simulink model "gm_sampleModel1400_5_sub"  (R2023a)
settings: Solver=VariableStepAuto  StartTime=0.0  StopTime=10.0  RelTol=1e-3
libraries: hdlsllib x1, simulink x1
settings Model: Creator=user1  LastModifiedBy=user1
settings OptimizationCC: BlockReduction=off  ConditionallyExecuteInputs=off
settings DebuggingCC: InheritedTsInSrcMsg=none

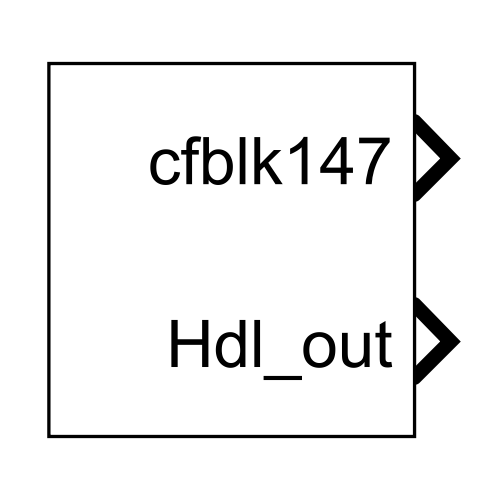
[thumbnail: Simulink's stored preview of the top-level diagram]
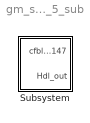
== system gm_sampleModel1400_5_sub ==
  Subsystem : Subsystem

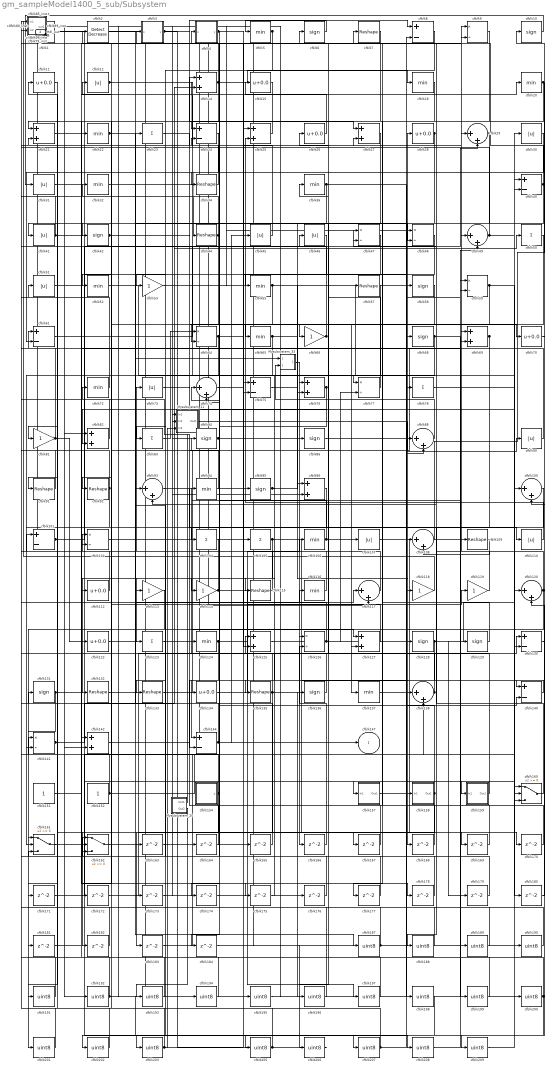
== system gm_sampleModel1400_5_sub/Subsystem ==
  Mysubsystem_11 : Subsystem
  Mysubsystem_20 : Subsystem
  Mysubsystem_33 : Subsystem
  cfblk1 : hdlsllib/Logic and Bit Operations/Bit Slice  lidx=7  ridx=0
  cfblk{6,10,42,58,68,84,86,95,128..129,131,136} (12 alike) : Signum
  cfblk{29,49,74,88,93,100,108,117,120,138} (10 alike) : Sum  Inputs=|++  OutDataTypeStr=uint8
  cfblk{8,24,40,61,75,101,130,140,144} (9 alike) : Sum  Inputs=+-  OutDataTypeStr=uint8
  cfblk{9,47..48,59,64,77,102,126,141} (9 alike) : Product  Inputs=*/  OutDataTypeStr=uint8  RndMeth=Zero  SaturateOnIntegerOverflow=on
  cfblk{23,50,78,83,104..105,123} (7 alike) : Sum  Inputs=+  OutDataTypeStr=uint8
  cfblk{5,18,20,22,32,36,52,55,65,72,94,106,116,124,137} (15 alike) : MinMax  OutDataTypeStr=uint8
  cfblk{12,30..31,41,45..46,51,73,90,107,110} (11 alike) : Abs  OutDataTypeStr=uint8  SaturateOnIntegerOverflow=off
  cfblk{7,34,44,57,91..92,109,115,132..133,135} (11 alike) : Reshape
  cfblk{11,15,26,28,70,112,122,134} (8 alike) : Bias  Bias=0.0  SaturateOnIntegerOverflow=off
  cfblk{53,66,81,113..114,118..119} (7 alike) : Gain  OutDataTypeStr=uint8
  cfblk{14,21,25,27,69,76,82,96,125,127,142} (11 alike) : Sum  OutDataTypeStr=uint8
  cfblk139_inst : Subsystem
  cfblk13_inst : Subsystem
  cfblk143_inst : Subsystem
  cfblk145_inst : Subsystem
  cfblk146_inst : Subsystem
  cfblk151 : Constant  OutDataTypeStr=uint8  SampleTime=-1
  cfblk152 : Constant  OutDataTypeStr=uint8  SampleTime=-1
  cfblk154 : Subsystem  mask(Counter Limited){uplimit=double(7), tsamp=double(-1)}
      mask prompts: uplimit "Simulink:masks:UpperLimit_MP"; tsamp "Simulink:masks:SampleTime_MP"
      mask help: Simulink:masks:CounterLimited_MD
      mask init:
      | nbits = double(8);
      | tsamp = double(-1);
      | uplimit = double(7);
  cfblk157 : Subsystem
  cfblk158 : Subsystem
  cfblk159 : Subsystem
  cfblk160 : Switch  OutDataTypeStr=uint8  SaturateOnIntegerOverflow=off  InputSameDT=off
  cfblk161 : Switch  OutDataTypeStr=uint8  SaturateOnIntegerOverflow=off  InputSameDT=off
  cfblk162 : Switch  OutDataTypeStr=uint8  SaturateOnIntegerOverflow=off  InputSameDT=off
  cfblk{163..184} (22 alike) : Delay  SampleTime=1
  cfblk16_inst : Subsystem
  cfblk17_inst : Subsystem
  cfblk{187..203,205..209} (22 alike) : DataTypeConversion  OutDataTypeStr=uint8  SaturateOnIntegerOverflow=off  RndMeth=Floor
  cfblk19_inst : Subsystem
  cfblk2 : simulink/Logic and Bit Operations/Detect Decrease  vinit=0.0  OutDataTypeStr=uint8
      settings: LibrarySourceBlock=|
      | hdlsllib/Logic and Bit
      | Operations/Detect
      | Decrease
  cfblk3 : Subsystem  mask(Compare To Zero){relop=<=, OutDataTypeStr=uint8, ZeroCross=on}
      mask prompts: relop "Simulink:masks:Operator_MP"; OutDataTypeStr "Simulink:masks:OutputDataType_MP"; ZeroCross "Simulink:masks:EnableZerocrossingDetection_MP"
      mask help: Simulink:masks:CompareToZero_MD
      mask init:
      | OutDataTypeStr = 'uint8';
      | ZeroCross = 'on';
      | blkName = 'sampleModel1400_5_sub/Subsystem/cfblk3';
      | relop = '<=';
      | setValue = 'fixdt(0, 8)';
      mask TypeOptions relop: == | ~= | < | <= | >= | >
      mask TypeOptions OutDataTypeStr: Simulink:masks:uint8 | Simulink:masks:boolean
      mask Callback ZeroCross: sl('zeroCrossEnable', gcbh);
      mask Display: disp([relop,' 0'])
  cfblk35_inst : Subsystem
  cfblk37_inst : Subsystem
  cfblk39_inst : Subsystem
  cfblk4 : Subsystem  mask(Compare To Constant){relop=<=, const=double(3), OutDataTypeStr=uint8, ZeroCross=on}
      mask prompts: relop "Simulink:masks:Operator_MP"; const "Simulink:masks:ConstantValue_MP"; OutDataTypeStr "Simulink:masks:OutputDataType_MP"; ZeroCross "Simulink:masks:EnableZerocrossingDetection_MP"
      mask help: Simulink:masks:CompareToConstant_MD
      mask init:
      | OutDataTypeStr = 'uint8';
      | ZeroCross = 'on';
      | blkName = 'sampleModel1400_5_sub/Subsystem/cfblk4';
      | const = double(3);
      | const_str = '3.0';
      | const_val = double(3);
      | relop = '<=';
      | setValue = 'fixdt(0, 8)';
      | str = '<= 3';
      mask TypeOptions relop: == | ~= | < | <= | >= | >
      mask TypeOptions OutDataTypeStr: Simulink:masks:uint8 | Simulink:masks:boolean
      mask Callback ZeroCross: sl('zeroCrossEnable', gcbh);
      mask Display: disp(str)
  cfblk43_inst : Subsystem
  cfblk54_inst : Subsystem
  cfblk60_inst : Subsystem
  cfblk62_inst : Subsystem
  cfblk67_inst : Subsystem
  cfblk71_inst : Subsystem
  cfblk79_inst : Subsystem
  cfblk80_inst : Subsystem
  cfblk85_inst : Subsystem
  cfblk98_inst : Subsystem
  cfblk99_inst : Subsystem
  cfblk147 : Outport  OutDataTypeStr=uint8  SampleTime=1  VectorParamsAs1DForOutWhenUnconnected=off
  Hdl_out : Outport  Port=2  OutDataTypeStr=uint8  SampleTime=1
  wires:
  Mysubsystem_11/1(Out1) -> cfblk168/1
  Mysubsystem_20/1(Out1) -> cfblk50/1
  Mysubsystem_20/2(Out2) -> cfblk193/1
  Mysubsystem_33/1(Out1) -> cfblk166/1
  cfblk1/1 -> cfblk205/1
  cfblk10/1 -> cfblk31/1
  cfblk100/1 -> cfblk188/1
  cfblk101/1 -> cfblk46/1, cfblk159/1(In1), cfblk157/1(In1)
  cfblk102/1 -> cfblk28/1
  cfblk104/1 -> cfblk132/1
  cfblk105/1 -> cfblk169/1, cfblk123/1
  cfblk106/1 -> cfblk6/1, cfblk4/1(u)
  cfblk107/1 -> cfblk170/1
  cfblk108/1 -> cfblk10/1
  cfblk109/1 -> cfblk108/2
  cfblk11/1 -> cfblk91/1
  cfblk110/1 -> cfblk25/2
  cfblk112/1 -> cfblk61/1
  cfblk113/1 -> cfblk201/1
  cfblk114/1 -> cfblk197/1, cfblk112/1
  cfblk115/1 -> cfblk60_inst/1(in1)
  cfblk116/1 -> cfblk99_inst/1(in1)
  cfblk117/1 -> cfblk73/1
  cfblk118/1 -> cfblk19_inst/2(in2)
  cfblk119/1 -> cfblk93/2
  cfblk12/1 -> cfblk76/1, cfblk44/1
  cfblk120/1 -> cfblk9/1, cfblk47/1, cfblk181/1
  cfblk122/1 -> cfblk116/1
  cfblk123/1 -> cfblk127/1
  cfblk124/1 -> cfblk144/1, cfblk119/1
  cfblk125/1 -> cfblk138/1
  cfblk126/1 -> cfblk71_inst/2(in2), cfblk77/2
  cfblk127/1 -> cfblk102/1
  cfblk128/1 -> cfblk30/1, cfblk144/2, cfblk179/1
  cfblk129/1 -> cfblk3/1(u)
  cfblk13_inst/1(out1) -> cfblk200/1
  cfblk130/1 -> cfblk207/1
  cfblk131/1 -> cfblk7/1, cfblk161/1
  cfblk132/1 -> cfblk94/1
  cfblk133/1 -> cfblk49/1
  cfblk134/1 -> cfblk106/1
  cfblk135/1 -> cfblk62_inst/1(in1), cfblk17_inst/2(in2), cfblk182/1, cfblk158/1(In1)
  cfblk136/1 -> cfblk11/1
  cfblk137/1 -> cfblk128/1
  cfblk138/1 -> cfblk99_inst/2(in2), cfblk12/1
  cfblk139_inst/1(out1) -> cfblk195/1
  cfblk14/1 -> cfblk43_inst/2(in2), cfblk21/1, cfblk18/1
  cfblk140/1 -> cfblk134/1
  cfblk141/1 -> cfblk51/1, cfblk14/2, cfblk23/1
  cfblk142/1 -> cfblk69/1
  cfblk143_inst/1(out1) -> cfblk101/2
  cfblk144/1 -> cfblk98_inst/2(in2), cfblk45/1
  cfblk145_inst/1(out1) -> cfblk95/1, cfblk142/2
  cfblk146_inst/1(out1) -> cfblk192/1
  cfblk15/1 -> cfblk64/2
  cfblk151/1 -> cfblk22/1
  cfblk152/1 -> cfblk35_inst/2(in2), cfblk108/1
  cfblk154/1(y) -> cfblk84/1, cfblk191/1, cfblk141/1
  cfblk157/1(Out1) -> cfblk140/2
  cfblk158/1(Out1) -> cfblk74/1, cfblk183/1
  cfblk159/1(Out1) -> cfblk36/1
  cfblk16_inst/1(out1) -> cfblk117/2
  cfblk160/1 -> cfblk62_inst/2(in2)
  cfblk161/1 -> cfblk175/1
  cfblk162/1 -> cfblk167/1
  cfblk163/1 -> cfblk138/2
  cfblk164/1 -> cfblk101/1
  cfblk165/1 -> cfblk37_inst/1(in1)
  cfblk166/1 -> cfblk126/2
  cfblk167/1 -> cfblk143_inst/2(in2)
  cfblk168/1 -> cfblk47/2
  cfblk169/1 -> cfblk80_inst/2(in2)
  cfblk17_inst/1(out1) -> cfblk165/1
  cfblk170/1 -> cfblk25/1
  cfblk171/1 -> cfblk40/2
  cfblk172/1 -> cfblk49/2
  cfblk173/1 -> cfblk59/2
  cfblk174/1 -> cfblk117/1
  cfblk175/1 -> cfblk125/1
  cfblk176/1 -> cfblk24/2
  cfblk177/1 -> cfblk39_inst/2(in2)
  cfblk178/1 -> cfblk93/1
  cfblk179/1 -> cfblk16_inst/1(in1)
  cfblk18/1 -> cfblk177/1
  cfblk180/1 -> cfblk120/2
  cfblk181/1 -> cfblk69/2
  cfblk182/1 -> cfblk145_inst/1(in1)
  cfblk183/1 -> cfblk8/2
  cfblk184/1 -> cfblk206/1
  cfblk187/1 -> cfblk90/1, cfblk131/1
  cfblk188/1 -> cfblk2/1
  cfblk189/1 -> cfblk79_inst/1(in1)
  cfblk19_inst/1(out1) -> cfblk58/1
  cfblk190/1 -> cfblk67_inst/1(in1)
  cfblk191/1 -> cfblk67_inst/2(in2)
  cfblk192/1 -> cfblk80_inst/1(in1), cfblk208/1
  cfblk193/1 -> cfblk146_inst/1(in1)
  cfblk194/1 -> cfblk146_inst/2(in2)
  cfblk195/1 -> cfblk136/1
  cfblk196/1 -> cfblk139_inst/1(in1)
  cfblk197/1 -> cfblk139_inst/2(in2)
  cfblk198/1 -> cfblk202/1
  cfblk199/1 -> cfblk32/1
  cfblk2/1 -> cfblk187/1
  cfblk20/1 -> cfblk140/1, cfblk52/1
  cfblk200/1 -> cfblk209/1, cfblk142/1
  cfblk201/1 -> cfblk13_inst/1(in1)
  cfblk202/1 -> cfblk13_inst/2(in2)
  cfblk203/1 -> cfblk79_inst/2(in2), cfblk9/2, Mysubsystem_11/3(In3)
  cfblk205/1 -> cfblk39_inst/1(in1), cfblk161/3
  cfblk206/1 -> cfblk1/1
  cfblk207/1 -> cfblk88/2, cfblk162/1
  cfblk208/1 -> cfblk130/1
  cfblk209/1 -> cfblk130/2
  cfblk21/1 -> cfblk178/1
  cfblk22/1 -> cfblk48/2, Mysubsystem_33/1(In1)
  cfblk23/1 -> cfblk77/1
  cfblk24/1 -> cfblk61/2
  cfblk25/1 -> cfblk24/1
  cfblk26/1 -> cfblk15/1
  cfblk27/1 -> cfblk196/1
  cfblk28/1 -> cfblk162/2, Mysubsystem_11/2(In2)
  cfblk29/1 -> cfblk41/1, Mysubsystem_11/1(In1)
  cfblk3/1(y) -> cfblk8/1, cfblk27/1
  cfblk30/1 -> cfblk92/1
  cfblk31/1 -> cfblk173/1
  cfblk32/1 -> cfblk198/1
  cfblk34/1 -> cfblk19_inst/1(in1)
  cfblk35_inst/1(out1) -> cfblk86/1, Hdl_out/1
  cfblk36/1 -> cfblk88/1, cfblk74/2
  cfblk37_inst/1(out1) -> cfblk124/1
  cfblk39_inst/1(out1) -> cfblk129/1, cfblk147/1
  cfblk4/1(y) -> cfblk75/1, cfblk184/1
  cfblk40/1 -> cfblk76/2, cfblk60_inst/2(in2), cfblk81/1
  cfblk41/1 -> cfblk75/2, cfblk17_inst/1(in1), cfblk78/1
  cfblk42/1 -> cfblk70/1, cfblk180/1
  cfblk43_inst/1(out1) -> cfblk176/1
  cfblk44/1 -> cfblk85_inst/2(in2), cfblk163/1
  cfblk45/1 -> cfblk14/1
  cfblk46/1 -> cfblk55/1
  cfblk47/1 -> cfblk126/1
  cfblk48/1 -> cfblk125/2
  cfblk49/1 -> cfblk40/1, cfblk145_inst/2(in2)
  cfblk5/1 -> cfblk34/1, cfblk133/1
  cfblk50/1 -> cfblk203/1
  cfblk51/1 -> cfblk20/1
  cfblk52/1 -> cfblk100/1
  cfblk53/1 -> cfblk27/2
  cfblk54_inst/1(out1) -> cfblk98_inst/1(in1)
  cfblk55/1 -> cfblk160/2, cfblk65/1
  cfblk57/1 -> cfblk135/1
  cfblk58/1 -> cfblk127/2
  cfblk59/1 -> cfblk160/1, cfblk172/1
  cfblk6/1 -> cfblk5/1
  cfblk60_inst/1(out1) -> cfblk190/1
  cfblk61/1 -> cfblk29/2
  cfblk62_inst/1(out1) -> cfblk54_inst/2(in2)
  cfblk64/1 -> cfblk66/1, cfblk171/1
  cfblk65/1 -> cfblk118/1, cfblk83/1
  cfblk66/1 -> cfblk85_inst/1(in1), cfblk16_inst/2(in2)
  cfblk67_inst/1(out1) -> cfblk189/1
  cfblk68/1 -> cfblk199/1, cfblk160/3, cfblk141/2
  cfblk69/1 -> cfblk162/3, cfblk104/1
  cfblk7/1 -> cfblk102/2
  cfblk70/1 -> cfblk100/2
  cfblk71_inst/1(out1) -> cfblk194/1
  cfblk72/1 -> cfblk37_inst/2(in2)
  cfblk73/1 -> cfblk137/1
  cfblk74/1 -> cfblk29/1
  cfblk75/1 -> cfblk96/1
  cfblk76/1 -> cfblk82/2, cfblk113/1
  cfblk77/1 -> cfblk26/1
  cfblk78/1 -> cfblk120/1
  cfblk79_inst/1(out1) -> cfblk48/1
  cfblk8/1 -> cfblk53/1
  cfblk80_inst/1(out1) -> cfblk107/1, cfblk105/1
  cfblk81/1 -> cfblk71_inst/1(in1), cfblk21/2, cfblk122/1
  cfblk82/1 -> cfblk43_inst/1(in1)
  cfblk83/1 -> cfblk64/1
  cfblk84/1 -> cfblk68/1, cfblk114/1
  cfblk85_inst/1(out1) -> cfblk164/1
  cfblk86/1 -> cfblk59/1
  cfblk88/1 -> Mysubsystem_33/2(In2)
  cfblk9/1 -> cfblk42/1
  cfblk90/1 -> cfblk54_inst/1(in1)
  cfblk91/1 -> cfblk143_inst/1(in1)
  cfblk92/1 -> cfblk35_inst/1(in1), cfblk161/2
  cfblk93/1 -> cfblk110/1
  cfblk94/1 -> cfblk72/1
  cfblk95/1 -> cfblk57/1, cfblk115/1
  cfblk96/1 -> cfblk174/1
  cfblk98_inst/1(out1) -> cfblk96/2, cfblk109/1
  cfblk99_inst/1(out1) -> cfblk82/1

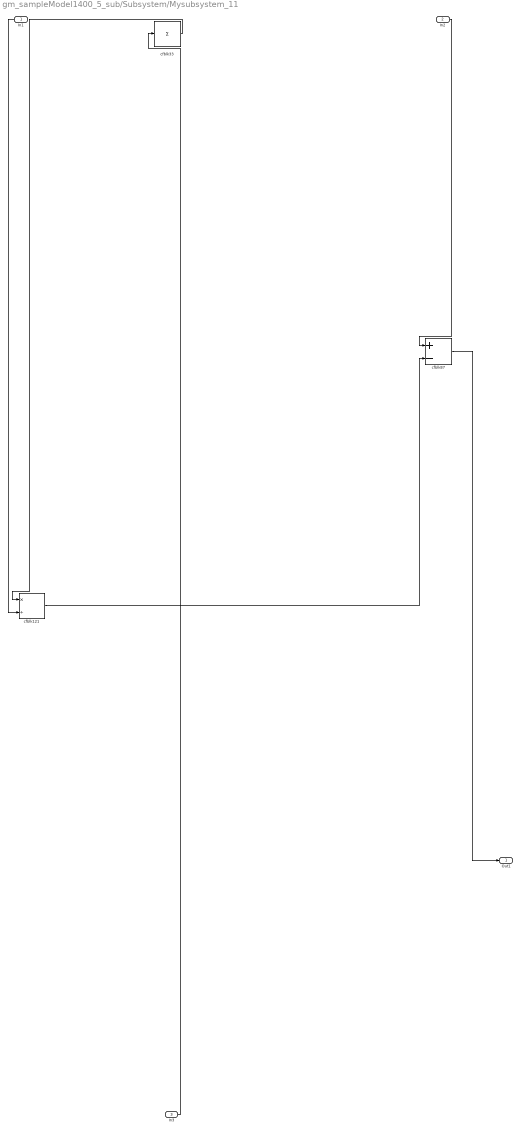
== system gm_sampleModel1400_5_sub/Subsystem/Mysubsystem_11 ==
  In1 : Inport  OutDataTypeStr=uint8  PortDimensions=1  SampleTime=1
  In2 : Inport  Port=2  OutDataTypeStr=uint8  PortDimensions=1  SampleTime=1
  In3 : Inport  Port=3  OutDataTypeStr=uint8  PortDimensions=1  SampleTime=1
  cfblk121 : Product  Inputs=*/  RndMeth=Zero  SaturateOnIntegerOverflow=on
  cfblk33 : Sum  Inputs=+
  cfblk87 : Sum  Inputs=+-
  Out1 : Outport  SampleTime=1
  wires:
  In1/1 -> cfblk121/2
  In2/1 -> cfblk87/1
  In3/1 -> cfblk33/1
  cfblk121/1 -> cfblk87/2
  cfblk33/1 -> cfblk121/1
  cfblk87/1 -> Out1/1

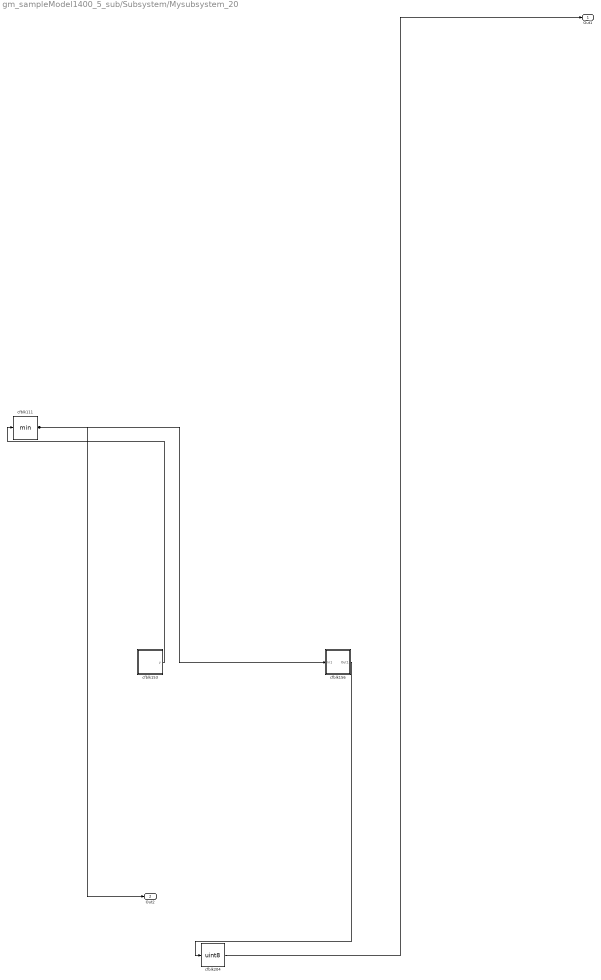
== system gm_sampleModel1400_5_sub/Subsystem/Mysubsystem_20 ==
  cfblk111 : MinMax
  cfblk153 : Subsystem  mask(Counter Free-Running){NumBits=double(16), tsamp=double(-1)}
      mask prompts: NumBits "Simulink:masks:NumberOfBits_MP"; tsamp "Simulink:masks:SampleTime_MP"
      mask help: Simulink:masks:CounterFreeRunning_MD
  cfblk156 : Subsystem
  cfblk204 : DataTypeConversion  OutDataTypeStr=uint8  SaturateOnIntegerOverflow=off  RndMeth=Floor
  Out1 : Outport  SampleTime=1
  Out2 : Outport  Port=2  SampleTime=1
  wires:
  cfblk111/1 -> cfblk156/1(In1), Out2/1
  cfblk153/1(y) -> cfblk111/1
  cfblk156/1(Out1) -> cfblk204/1
  cfblk204/1 -> Out1/1

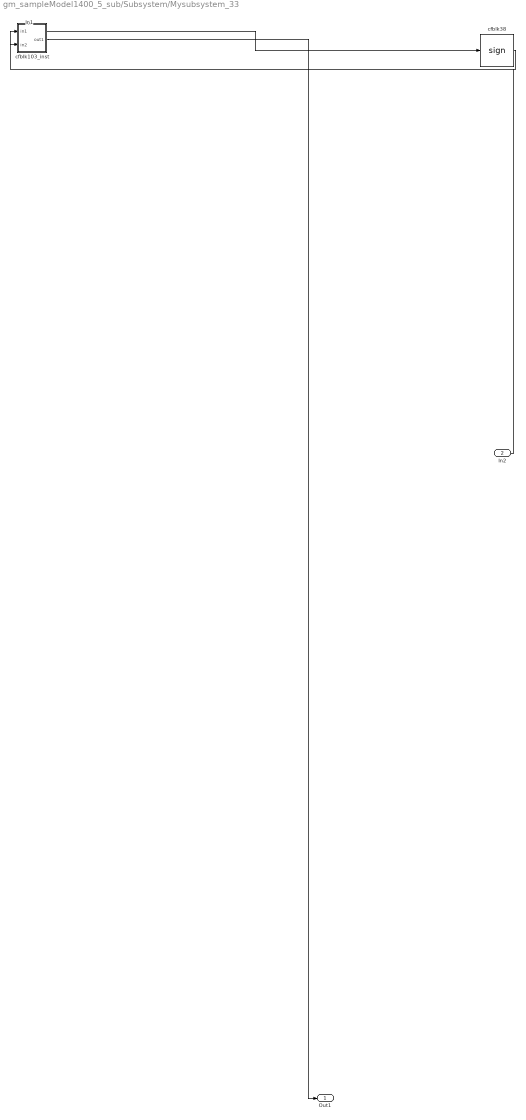
== system gm_sampleModel1400_5_sub/Subsystem/Mysubsystem_33 ==
  In1 : Inport  OutDataTypeStr=uint8  PortDimensions=1  SampleTime=1
  In2 : Inport  Port=2  OutDataTypeStr=uint8  PortDimensions=1  SampleTime=1
  cfblk103_inst : Subsystem
  cfblk38 : Signum
  Out1 : Outport  SampleTime=1
  wires:
  In1/1 -> cfblk38/1
  In2/1 -> cfblk103_inst/1(in1)
  cfblk103_inst/1(out1) -> Out1/1
  cfblk38/1 -> cfblk103_inst/2(in2)

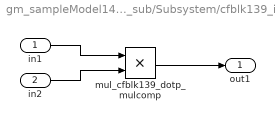
== system gm_sampleModel1400_5_sub/Subsystem/cfblk139_inst ==
  in1 : Inport  OutDataTypeStr=uint8  SampleTime=1
  in2 : Inport  Port=2  OutDataTypeStr=uint8  SampleTime=1
  mul_cfblk139_dotp_mulcomp : Product  Inputs=**  OutDataTypeStr=uint8  SampleTime=1
  out1 : Outport  OutDataTypeStr=uint8  SampleTime=1
  wires:
  in1/1 -> mul_cfblk139_dotp_mulcomp/1
  in2/1 -> mul_cfblk139_dotp_mulcomp/2
  mul_cfblk139_dotp_mulcomp/1 -> out1/1

== system gm_sampleModel1400_5_sub/Subsystem/cfblk13_inst ==
  in1 : Inport  OutDataTypeStr=uint8  SampleTime=1
  in2 : Inport  Port=2  OutDataTypeStr=uint8  SampleTime=1
  mul_cfblk13_dotp_mulcomp : Product  Inputs=**  OutDataTypeStr=uint8  SampleTime=1
  out1 : Outport  OutDataTypeStr=uint8  SampleTime=1
  wires:
  in1/1 -> mul_cfblk13_dotp_mulcomp/1
  in2/1 -> mul_cfblk13_dotp_mulcomp/2
  mul_cfblk13_dotp_mulcomp/1 -> out1/1

== system gm_sampleModel1400_5_sub/Subsystem/cfblk143_inst ==
  in1 : Inport  OutDataTypeStr=uint8  SampleTime=1
  in2 : Inport  Port=2  OutDataTypeStr=uint8  SampleTime=1
  mul_cfblk143_dotp_mulcomp : Product  Inputs=**  OutDataTypeStr=uint8  SampleTime=1
  out1 : Outport  OutDataTypeStr=uint8  SampleTime=1
  wires:
  in1/1 -> mul_cfblk143_dotp_mulcomp/1
  in2/1 -> mul_cfblk143_dotp_mulcomp/2
  mul_cfblk143_dotp_mulcomp/1 -> out1/1

== system gm_sampleModel1400_5_sub/Subsystem/cfblk145_inst ==
  in1 : Inport  OutDataTypeStr=uint8  SampleTime=1
  in2 : Inport  Port=2  OutDataTypeStr=uint8  SampleTime=1
  mul_cfblk145_dotp_mulcomp : Product  Inputs=**  OutDataTypeStr=uint8  SampleTime=1
  out1 : Outport  OutDataTypeStr=uint8  SampleTime=1
  wires:
  in1/1 -> mul_cfblk145_dotp_mulcomp/1
  in2/1 -> mul_cfblk145_dotp_mulcomp/2
  mul_cfblk145_dotp_mulcomp/1 -> out1/1

== system gm_sampleModel1400_5_sub/Subsystem/cfblk146_inst ==
  in1 : Inport  OutDataTypeStr=uint8  SampleTime=1
  in2 : Inport  Port=2  OutDataTypeStr=uint8  SampleTime=1
  mul_cfblk146_dotp_mulcomp : Product  Inputs=**  OutDataTypeStr=uint8  SampleTime=1
  out1 : Outport  OutDataTypeStr=uint8  SampleTime=1
  wires:
  in1/1 -> mul_cfblk146_dotp_mulcomp/1
  in2/1 -> mul_cfblk146_dotp_mulcomp/2
  mul_cfblk146_dotp_mulcomp/1 -> out1/1

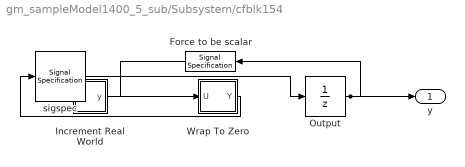
== system gm_sampleModel1400_5_sub/Subsystem/cfblk154 ==
  Force to be scalar : SignalSpecification  DisableCoverage=on  Dimensions=1
  Increment Real World : Subsystem  mask(Real World Value Increment){}
      mask help: Simulink:masks:RealWorldValueIncrement_MD
      mask Display: disp('V++')
  Output : UnitDelay  InitialCondition=0.0  SampleTime=tsamp  HasFrameUpgradeWarning=on
  Wrap To Zero : Subsystem  mask(Wrap To Zero){Threshold=double(7)}
      mask prompts: Threshold "Simulink:masks:Threshold_MP"
      mask help: Simulink:masks:WrapToZero_MD
  sigspec : SignalSpecification  OutDataTypeStr=uint8  Dimensions=1
  y : Outport  SampleTime=1
  wires:
  Force to be scalar/1 -> Increment Real World/1(u)
  Increment Real World/1(y) -> Wrap To Zero/1(U)
  Output/1 -> Force to be scalar/1, y/1
  Wrap To Zero/1(Y) -> sigspec/1
  sigspec/1 -> Output/1

== system gm_sampleModel1400_5_sub/Subsystem/cfblk157 ==
  In1 : Inport  OutDataTypeStr=uint8  PortDimensions=1  SampleTime=1
  Out1 : Outport  SampleTime=1
  wires:
  In1/1 -> Out1/1

== system gm_sampleModel1400_5_sub/Subsystem/cfblk158 ==
  In1 : Inport  OutDataTypeStr=uint8  PortDimensions=1  SampleTime=1
  Out1 : Outport  SampleTime=1
  wires:
  In1/1 -> Out1/1

== system gm_sampleModel1400_5_sub/Subsystem/cfblk159 ==
  In1 : Inport  OutDataTypeStr=uint8  PortDimensions=1  SampleTime=1
  Out1 : Outport  SampleTime=1
  wires:
  In1/1 -> Out1/1

== system gm_sampleModel1400_5_sub/Subsystem/cfblk16_inst ==
  in1 : Inport  OutDataTypeStr=uint8  SampleTime=1
  in2 : Inport  Port=2  OutDataTypeStr=uint8  SampleTime=1
  mul_cfblk16_dotp_mulcomp : Product  Inputs=**  OutDataTypeStr=uint8  SampleTime=1
  out1 : Outport  OutDataTypeStr=uint8  SampleTime=1
  wires:
  in1/1 -> mul_cfblk16_dotp_mulcomp/1
  in2/1 -> mul_cfblk16_dotp_mulcomp/2
  mul_cfblk16_dotp_mulcomp/1 -> out1/1

== system gm_sampleModel1400_5_sub/Subsystem/cfblk17_inst ==
  in1 : Inport  OutDataTypeStr=uint8  SampleTime=1
  in2 : Inport  Port=2  OutDataTypeStr=uint8  SampleTime=1
  mul_cfblk17_dotp_mulcomp : Product  Inputs=**  OutDataTypeStr=uint8  SampleTime=1
  out1 : Outport  OutDataTypeStr=uint8  SampleTime=1
  wires:
  in1/1 -> mul_cfblk17_dotp_mulcomp/1
  in2/1 -> mul_cfblk17_dotp_mulcomp/2
  mul_cfblk17_dotp_mulcomp/1 -> out1/1

== system gm_sampleModel1400_5_sub/Subsystem/cfblk19_inst ==
  in1 : Inport  OutDataTypeStr=uint8  SampleTime=1
  in2 : Inport  Port=2  OutDataTypeStr=uint8  SampleTime=1
  mul_cfblk19_dotp_mulcomp : Product  Inputs=**  OutDataTypeStr=uint8  SampleTime=1
  out1 : Outport  OutDataTypeStr=uint8  SampleTime=1
  wires:
  in1/1 -> mul_cfblk19_dotp_mulcomp/1
  in2/1 -> mul_cfblk19_dotp_mulcomp/2
  mul_cfblk19_dotp_mulcomp/1 -> out1/1

== system gm_sampleModel1400_5_sub/Subsystem/cfblk3 ==
  u : Inport  OutDataTypeStr=uint8  SampleTime=1
  Compare : RelationalOperator  Operator=<=  OutDataTypeStr=fixdt(0, 8)
  Constant : Constant  DisableCoverage=on  Value=0  OutDataTypeStr=Inherit: Inherit via back propagation  SampleTime=-1  PreserveConstantTs=on
  y : Outport  SampleTime=1
  wires:
  u/1 -> Compare/1
  Compare/1 -> y/1
  Constant/1 -> Compare/2

== system gm_sampleModel1400_5_sub/Subsystem/cfblk35_inst ==
  in1 : Inport  OutDataTypeStr=uint8  SampleTime=1
  in2 : Inport  Port=2  OutDataTypeStr=uint8  SampleTime=1
  mul_cfblk35_dotp_mulcomp : Product  Inputs=**  OutDataTypeStr=uint8  SampleTime=1
  out1 : Outport  OutDataTypeStr=uint8  SampleTime=1
  wires:
  in1/1 -> mul_cfblk35_dotp_mulcomp/1
  in2/1 -> mul_cfblk35_dotp_mulcomp/2
  mul_cfblk35_dotp_mulcomp/1 -> out1/1

== system gm_sampleModel1400_5_sub/Subsystem/cfblk37_inst ==
  in1 : Inport  OutDataTypeStr=uint8  SampleTime=1
  in2 : Inport  Port=2  OutDataTypeStr=uint8  SampleTime=1
  mul_cfblk37_dotp_mulcomp : Product  Inputs=**  OutDataTypeStr=uint8  SampleTime=1
  out1 : Outport  OutDataTypeStr=uint8  SampleTime=1
  wires:
  in1/1 -> mul_cfblk37_dotp_mulcomp/1
  in2/1 -> mul_cfblk37_dotp_mulcomp/2
  mul_cfblk37_dotp_mulcomp/1 -> out1/1

== system gm_sampleModel1400_5_sub/Subsystem/cfblk39_inst ==
  in1 : Inport  OutDataTypeStr=uint8  SampleTime=1
  in2 : Inport  Port=2  OutDataTypeStr=uint8  SampleTime=1
  mul_cfblk39_dotp_mulcomp : Product  Inputs=**  OutDataTypeStr=uint8  SampleTime=1
  out1 : Outport  OutDataTypeStr=uint8  SampleTime=1
  wires:
  in1/1 -> mul_cfblk39_dotp_mulcomp/1
  in2/1 -> mul_cfblk39_dotp_mulcomp/2
  mul_cfblk39_dotp_mulcomp/1 -> out1/1

== system gm_sampleModel1400_5_sub/Subsystem/cfblk4 ==
  u : Inport  OutDataTypeStr=uint8  SampleTime=1
  Compare : RelationalOperator  Operator=<=  OutDataTypeStr=fixdt(0, 8)
  Constant : Constant  DisableCoverage=on  Value=const  OutDataTypeStr=Inherit: Inherit via back propagation  SampleTime=-1
  y : Outport  SampleTime=1
  wires:
  u/1 -> Compare/1
  Compare/1 -> y/1
  Constant/1 -> Compare/2

== system gm_sampleModel1400_5_sub/Subsystem/cfblk43_inst ==
  in1 : Inport  OutDataTypeStr=uint8  SampleTime=1
  in2 : Inport  Port=2  OutDataTypeStr=uint8  SampleTime=1
  mul_cfblk43_dotp_mulcomp : Product  Inputs=**  OutDataTypeStr=uint8  SampleTime=1
  out1 : Outport  OutDataTypeStr=uint8  SampleTime=1
  wires:
  in1/1 -> mul_cfblk43_dotp_mulcomp/1
  in2/1 -> mul_cfblk43_dotp_mulcomp/2
  mul_cfblk43_dotp_mulcomp/1 -> out1/1

== system gm_sampleModel1400_5_sub/Subsystem/cfblk54_inst ==
  in1 : Inport  OutDataTypeStr=uint8  SampleTime=1
  in2 : Inport  Port=2  OutDataTypeStr=uint8  SampleTime=1
  mul_cfblk54_dotp_mulcomp : Product  Inputs=**  OutDataTypeStr=uint8  SampleTime=1
  out1 : Outport  OutDataTypeStr=uint8  SampleTime=1
  wires:
  in1/1 -> mul_cfblk54_dotp_mulcomp/1
  in2/1 -> mul_cfblk54_dotp_mulcomp/2
  mul_cfblk54_dotp_mulcomp/1 -> out1/1

== system gm_sampleModel1400_5_sub/Subsystem/cfblk60_inst ==
  in1 : Inport  OutDataTypeStr=uint8  SampleTime=1
  in2 : Inport  Port=2  OutDataTypeStr=uint8  SampleTime=1
  mul_cfblk60_dotp_mulcomp : Product  Inputs=**  OutDataTypeStr=uint8  SampleTime=1
  out1 : Outport  OutDataTypeStr=uint8  SampleTime=1
  wires:
  in1/1 -> mul_cfblk60_dotp_mulcomp/1
  in2/1 -> mul_cfblk60_dotp_mulcomp/2
  mul_cfblk60_dotp_mulcomp/1 -> out1/1

== system gm_sampleModel1400_5_sub/Subsystem/cfblk62_inst ==
  in1 : Inport  OutDataTypeStr=uint8  SampleTime=1
  in2 : Inport  Port=2  OutDataTypeStr=uint8  SampleTime=1
  mul_cfblk62_dotp_mulcomp : Product  Inputs=**  OutDataTypeStr=uint8  SampleTime=1
  out1 : Outport  OutDataTypeStr=uint8  SampleTime=1
  wires:
  in1/1 -> mul_cfblk62_dotp_mulcomp/1
  in2/1 -> mul_cfblk62_dotp_mulcomp/2
  mul_cfblk62_dotp_mulcomp/1 -> out1/1

== system gm_sampleModel1400_5_sub/Subsystem/cfblk67_inst ==
  in1 : Inport  OutDataTypeStr=uint8  SampleTime=1
  in2 : Inport  Port=2  OutDataTypeStr=uint8  SampleTime=1
  mul_cfblk67_dotp_mulcomp : Product  Inputs=**  OutDataTypeStr=uint8  SampleTime=1
  out1 : Outport  OutDataTypeStr=uint8  SampleTime=1
  wires:
  in1/1 -> mul_cfblk67_dotp_mulcomp/1
  in2/1 -> mul_cfblk67_dotp_mulcomp/2
  mul_cfblk67_dotp_mulcomp/1 -> out1/1

== system gm_sampleModel1400_5_sub/Subsystem/cfblk71_inst ==
  in1 : Inport  OutDataTypeStr=uint8  SampleTime=1
  in2 : Inport  Port=2  OutDataTypeStr=uint8  SampleTime=1
  mul_cfblk71_dotp_mulcomp : Product  Inputs=**  OutDataTypeStr=uint8  SampleTime=1
  out1 : Outport  OutDataTypeStr=uint8  SampleTime=1
  wires:
  in1/1 -> mul_cfblk71_dotp_mulcomp/1
  in2/1 -> mul_cfblk71_dotp_mulcomp/2
  mul_cfblk71_dotp_mulcomp/1 -> out1/1

== system gm_sampleModel1400_5_sub/Subsystem/cfblk79_inst ==
  in1 : Inport  OutDataTypeStr=uint8  SampleTime=1
  in2 : Inport  Port=2  OutDataTypeStr=uint8  SampleTime=1
  mul_cfblk79_dotp_mulcomp : Product  Inputs=**  OutDataTypeStr=uint8  SampleTime=1
  out1 : Outport  OutDataTypeStr=uint8  SampleTime=1
  wires:
  in1/1 -> mul_cfblk79_dotp_mulcomp/1
  in2/1 -> mul_cfblk79_dotp_mulcomp/2
  mul_cfblk79_dotp_mulcomp/1 -> out1/1

== system gm_sampleModel1400_5_sub/Subsystem/cfblk80_inst ==
  in1 : Inport  OutDataTypeStr=uint8  SampleTime=1
  in2 : Inport  Port=2  OutDataTypeStr=uint8  SampleTime=1
  mul_cfblk80_dotp_mulcomp : Product  Inputs=**  OutDataTypeStr=uint8  SampleTime=1
  out1 : Outport  OutDataTypeStr=uint8  SampleTime=1
  wires:
  in1/1 -> mul_cfblk80_dotp_mulcomp/1
  in2/1 -> mul_cfblk80_dotp_mulcomp/2
  mul_cfblk80_dotp_mulcomp/1 -> out1/1

== system gm_sampleModel1400_5_sub/Subsystem/cfblk85_inst ==
  in1 : Inport  OutDataTypeStr=uint8  SampleTime=1
  in2 : Inport  Port=2  OutDataTypeStr=uint8  SampleTime=1
  mul_cfblk85_dotp_mulcomp : Product  Inputs=**  OutDataTypeStr=uint8  SampleTime=1
  out1 : Outport  OutDataTypeStr=uint8  SampleTime=1
  wires:
  in1/1 -> mul_cfblk85_dotp_mulcomp/1
  in2/1 -> mul_cfblk85_dotp_mulcomp/2
  mul_cfblk85_dotp_mulcomp/1 -> out1/1

== system gm_sampleModel1400_5_sub/Subsystem/cfblk98_inst ==
  in1 : Inport  OutDataTypeStr=uint8  SampleTime=1
  in2 : Inport  Port=2  OutDataTypeStr=uint8  SampleTime=1
  mul_cfblk98_dotp_mulcomp : Product  Inputs=**  OutDataTypeStr=uint8  SampleTime=1
  out1 : Outport  OutDataTypeStr=uint8  SampleTime=1
  wires:
  in1/1 -> mul_cfblk98_dotp_mulcomp/1
  in2/1 -> mul_cfblk98_dotp_mulcomp/2
  mul_cfblk98_dotp_mulcomp/1 -> out1/1

== system gm_sampleModel1400_5_sub/Subsystem/cfblk99_inst ==
  in1 : Inport  OutDataTypeStr=uint8  SampleTime=1
  in2 : Inport  Port=2  OutDataTypeStr=uint8  SampleTime=1
  mul_cfblk99_dotp_mulcomp : Product  Inputs=**  OutDataTypeStr=uint8  SampleTime=1
  out1 : Outport  OutDataTypeStr=uint8  SampleTime=1
  wires:
  in1/1 -> mul_cfblk99_dotp_mulcomp/1
  in2/1 -> mul_cfblk99_dotp_mulcomp/2
  mul_cfblk99_dotp_mulcomp/1 -> out1/1

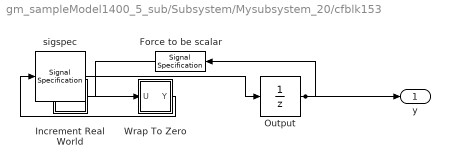
== system gm_sampleModel1400_5_sub/Subsystem/Mysubsystem_20/cfblk153 ==
  Force to be scalar : SignalSpecification  DisableCoverage=on  Dimensions=1
  Increment Real World : Subsystem  mask(Real World Value Increment){}
      mask help: Simulink:masks:RealWorldValueIncrement_MD
      mask Display: disp('V++')
  Output : UnitDelay  InitialCondition=0.0  SampleTime=tsamp  HasFrameUpgradeWarning=on
  Wrap To Zero : Subsystem  mask(Wrap To Zero){Threshold=double(65535)}
      mask prompts: Threshold "Simulink:masks:Threshold_MP"
      mask help: Simulink:masks:WrapToZero_MD
  sigspec : SignalSpecification  OutDataTypeStr=uint16  Dimensions=1
  y : Outport  SampleTime=1
  wires:
  Force to be scalar/1 -> Increment Real World/1(u)
  Increment Real World/1(y) -> Wrap To Zero/1(U)
  Output/1 -> Force to be scalar/1, y/1
  Wrap To Zero/1(Y) -> sigspec/1
  sigspec/1 -> Output/1

== system gm_sampleModel1400_5_sub/Subsystem/Mysubsystem_20/cfblk156 ==
  In1 : Inport  OutDataTypeStr=uint16  PortDimensions=1  SampleTime=1
  Out1 : Outport  SampleTime=1
  wires:
  In1/1 -> Out1/1

== system gm_sampleModel1400_5_sub/Subsystem/Mysubsystem_33/cfblk103_inst ==
  in1 : Inport  OutDataTypeStr=uint8  SampleTime=1
  in2 : Inport  Port=2  OutDataTypeStr=uint8  SampleTime=1
  mul_cfblk103_dotp_mulcomp : Product  Inputs=**  OutDataTypeStr=uint16  SampleTime=1
  out1 : Outport  OutDataTypeStr=uint16  SampleTime=1
  wires:
  in1/1 -> mul_cfblk103_dotp_mulcomp/1
  in2/1 -> mul_cfblk103_dotp_mulcomp/2
  mul_cfblk103_dotp_mulcomp/1 -> out1/1

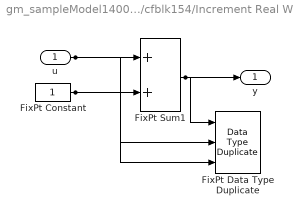
== system gm_sampleModel1400_5_sub/Subsystem/cfblk154/Increment Real World ==
  u : Inport  OutDataTypeStr=uint8  SampleTime=1
  FixPt Constant : Constant  DisableCoverage=on  OutDataTypeStr=Inherit: Inherit via back propagation  SampleTime=-1
  FixPt Data Type Duplicate : DataTypeDuplicate  DisableCoverage=on  NumInputPorts=3
  FixPt Sum1 : Sum  InputSameDT=on  OutDataTypeStr=Inherit: Inherit via back propagation  LockScale=on
  y : Outport  SampleTime=1
  wires:
  u/1 -> FixPt Sum1/1, FixPt Data Type Duplicate/2
  FixPt Constant/1 -> FixPt Sum1/2, FixPt Data Type Duplicate/3
  FixPt Sum1/1 -> FixPt Data Type Duplicate/1, y/1

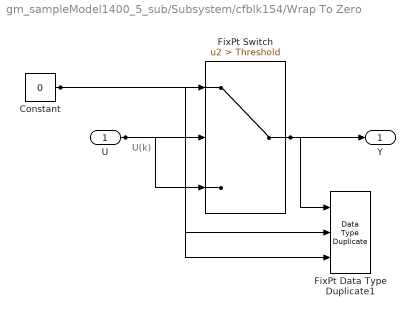
== system gm_sampleModel1400_5_sub/Subsystem/cfblk154/Wrap To Zero ==
  note: U(k)
  U : Inport  OutDataTypeStr=uint8  SampleTime=1
  Constant : Constant  DisableCoverage=on  Value=0  OutDataTypeStr=Inherit: Inherit via back propagation  SampleTime=-1
  FixPt Data Type Duplicate1 : DataTypeDuplicate  DisableCoverage=on  NumInputPorts=3
  FixPt Switch : Switch  Criteria=u2 > Threshold  Threshold=Threshold  OutDataTypeStr=Inherit: Inherit via back propagation  ZeroCross=off  SaturateOnIntegerOverflow=off  InputSameDT=off
  Y : Outport  SampleTime=1
  wires:
  U/1 -> FixPt Switch/3, FixPt Switch/2, FixPt Data Type Duplicate1/2
  Constant/1 -> FixPt Switch/1, FixPt Data Type Duplicate1/3
  FixPt Switch/1 -> FixPt Data Type Duplicate1/1, Y/1

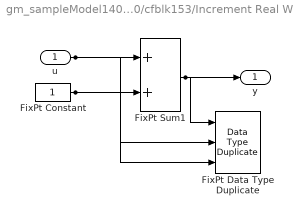
== system gm_sampleModel1400_5_sub/Subsystem/Mysubsystem_20/cfblk153/Increment Real World ==
  u : Inport  OutDataTypeStr=uint16  SampleTime=1
  FixPt Constant : Constant  DisableCoverage=on  OutDataTypeStr=Inherit: Inherit via back propagation  SampleTime=-1
  FixPt Data Type Duplicate : DataTypeDuplicate  DisableCoverage=on  NumInputPorts=3
  FixPt Sum1 : Sum  InputSameDT=on  OutDataTypeStr=Inherit: Inherit via back propagation  LockScale=on
  y : Outport  SampleTime=1
  wires:
  u/1 -> FixPt Sum1/1, FixPt Data Type Duplicate/2
  FixPt Constant/1 -> FixPt Sum1/2, FixPt Data Type Duplicate/3
  FixPt Sum1/1 -> FixPt Data Type Duplicate/1, y/1

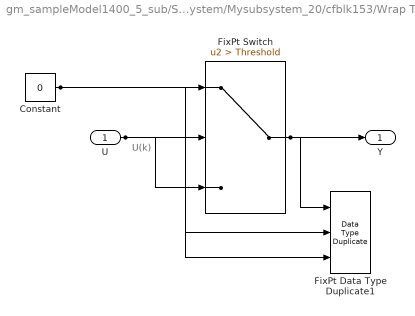
== system gm_sampleModel1400_5_sub/Subsystem/Mysubsystem_20/cfblk153/Wrap To Zero ==
  note: U(k)
  U : Inport  OutDataTypeStr=uint16  SampleTime=1
  Constant : Constant  DisableCoverage=on  Value=0  OutDataTypeStr=Inherit: Inherit via back propagation  SampleTime=-1
  FixPt Data Type Duplicate1 : DataTypeDuplicate  DisableCoverage=on  NumInputPorts=3
  FixPt Switch : Switch  Criteria=u2 > Threshold  Threshold=Threshold  OutDataTypeStr=Inherit: Inherit via back propagation  ZeroCross=off  SaturateOnIntegerOverflow=off  InputSameDT=off
  Y : Outport  SampleTime=1
  wires:
  U/1 -> FixPt Switch/3, FixPt Switch/2, FixPt Data Type Duplicate1/2
  Constant/1 -> FixPt Switch/1, FixPt Data Type Duplicate1/3
  FixPt Switch/1 -> FixPt Data Type Duplicate1/1, Y/1
